simulink subsystem "controller"  (R2024b)
settings: Solver=VariableStepAuto  StartTime=0.0  StopTime=10.0  RelTol=1e-3
values from neighbouring files (symbols this model uses):
  const_brake = 0    [selftest.m]
settings Model: Creator=yevge  LastModifiedBy=yevge

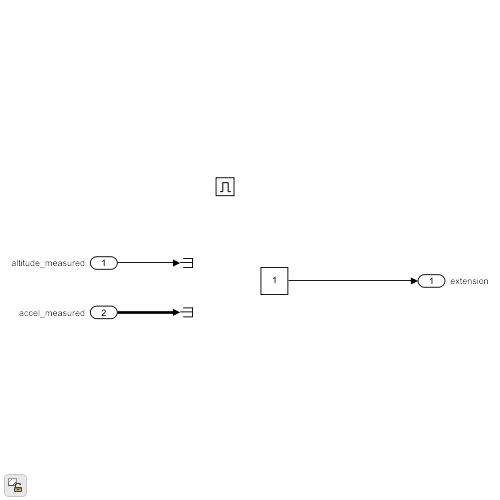
[thumbnail: Simulink's stored preview of the top-level diagram]
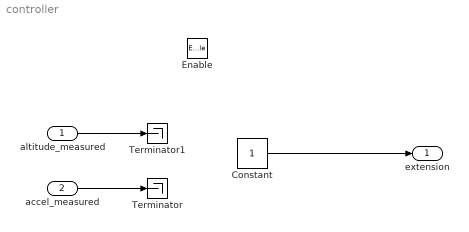
== system controller ==
  altitude_measured : Inport  Unit=m  PortDimensions=1
  accel_measured : Inport  Port=2  Unit=m/s^2  PortDimensions=[2 1]
  Enable : EnablePort  StatesWhenEnabling=reset
  Constant : Constant
  Terminator : Terminator
  Terminator1 : Terminator
  extension : Outport  OutMin=0  OutMax=1  Unit=1  PortDimensions=1  InitialOutput=const_brake
  wires:
  accel_measured/1 -> Terminator/1
  altitude_measured/1 -> Terminator1/1
  Constant/1 -> extension/1
